simulink model "ultra"  (R2015a)
settings: Solver=ode3  StartTime=0.0  StopTime=inf  RelTol=1e-3
values from neighbouring files (symbols this model uses):
  dis_cm = distance*100    [testbench_intial.m]
libraries: legoev3lib x2
settings Model: SimulationMode=external  CovMetricSettings=dwe  CovHtmlReporting=off  covSaveCumulativeToWorkspaceVar=off  CovSaveSingleToWorkspaceVar=off  CovExternalEMLEnable=on  ExtModeTrigDuration=2  Creator=karanverma  LastModifiedBy=Keshav
settings OptimizationCC: OptimizeModelRefInitCode=on  LifeSpan=1
settings DebuggingCC: UnderspecifiedInitializationDetection=Classic  MergeDetectMultiDrivingBlocksExec=none
settings HardwareCC: ProdLargestAtomicInteger=Long  ProdLargestAtomicFloat=Float  ProdEndianess=LittleEndian  ProdHWDeviceType=ARM Compatible->ARM 9
settings RTWCC: SystemTargetFile=realtime.tlc  GenerateMakefile=off  TemplateMakefile=realtime.tmf  Description=Run on Target Hardware  RTWVerbose=off
settings ERTTargetCC: CombineOutputUpdateFcns=off  ExtMode=on  ExtModeMexArgs='192.168.0.104' 0 17725  ERTSrcFileBannerTemplate=realtime_code_template.cgt  ERTHdrFileBannerTemplate=realtime_code_template.cgt  ERTDataSrcFileTemplate=realtime_code_template.cgt  ERTDataHdrFileTemplate=realtime_code_template.cgt  ERTCustomFileTemplate=realtime_file_process.tlc

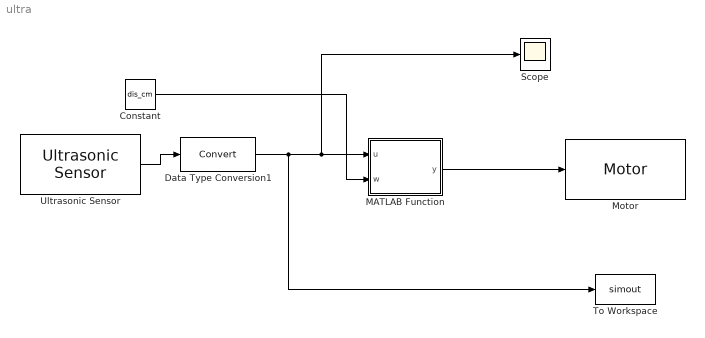
== system ultra ==
  Constant : Constant  Value=dis_cm
  Data Type Conversion1 : DataTypeConversion
  MATLAB Function : MATLAB Function  TreatAsAtomicUnit=on
  Motor : legoev3lib/Motor  sportNumber=A  sstopAction=Brake
  Scope : Scope
      settings: YMin=2.5  YMax=45
  To Workspace : ToWorkspace  VariableName=simout  SampleTime=-1
  Ultrasonic Sensor : legoev3lib/Ultrasonic Sensor  PortNumber=1  sampleTime=0.1
  wires:
  MATLAB Function/1(y) -> Motor/1
  Ultrasonic Sensor/1 -> Data Type Conversion1/1
  Data Type Conversion1/1 -> To Workspace/1, MATLAB Function/1(u), Scope/1
  Constant/1 -> MATLAB Function/2(w)

== matlab function ultra/MATLAB Function ==
  data: u input; y output; w input
function y = fcn(u,w)
y = 30;
x=w;
if((u-x)>30)|| ((u-x)<-30)
    y = 0;
elseif(u>4)&&(u<=20)
    y = 40;
end
end
